simulink model "measurement_setup"  (R2021b)
settings: Solver=VariableStepAuto  StartTime=0.0  StopTime=sim_duration  MaxStep=1e-5  RelTol=1e-7
values from neighbouring files (symbols this model uses):
  f_gen = 6000    [amplitude_test_simulation.m]    (also in dibs_simulation.m; noise_simulation.m = params.generation_freq; prbs_simulation.m = 3000; simulate.m = params.generation_freq)
  Fs = 4*f_gen    (= 24000)    [amplitude_test_simulation.m]    (also in dibs_simulation.m; noise_simulation.m = params.sampling_freq; prbs_simulation.m = 12000; simulate.m = params.sampling_freq)
libraries: cstblocks x1
settings Model: Creator=stdnt  LastModifiedBy=stdnt
settings DataIOCC: ReturnWorkspaceOutputs=off

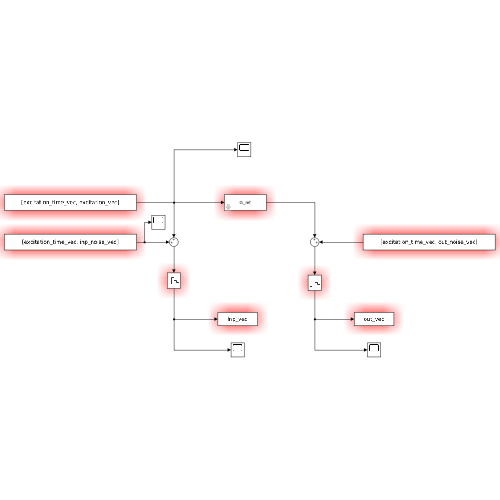
[thumbnail: Simulink's stored preview of the top-level diagram]
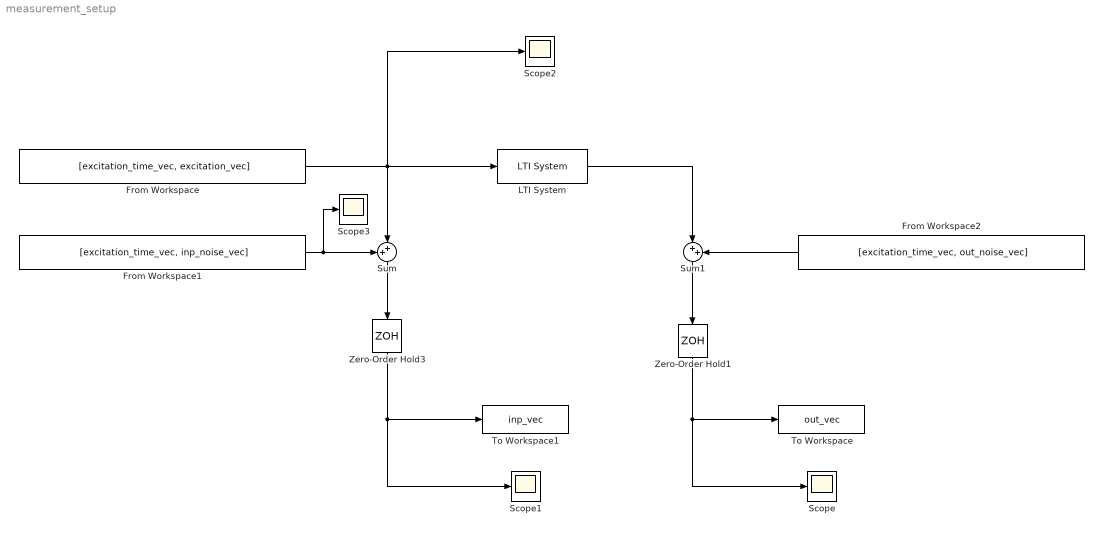
== system measurement_setup ==
  From Workspace : FromWorkspace  VariableName=[excitation_time_vec, excitation_vec]  SampleTime=1/f_gen  Interpolate=off  ZeroCross=off  OutputAfterFinalValue=Holding final value
  From Workspace1 : FromWorkspace  VariableName=[excitation_time_vec, inp_noise_vec]  SampleTime=1/f_gen  Interpolate=off  ZeroCross=off  OutputAfterFinalValue=Holding final value
  From Workspace2 : FromWorkspace  VariableName=[excitation_time_vec, out_noise_vec]  SampleTime=1/f_gen  Interpolate=off  ZeroCross=off  OutputAfterFinalValue=Holding final value
  LTI System : cstblocks/LTI System  sys=G_ref  IC=[]
  Scope{,1..3} (4 alike) : Scope
  Sum : Sum  Inputs=++|
  Sum1 : Sum  Inputs=|++
  To Workspace : ToWorkspace  VariableName=out_vec  SampleTime=1/Fs
  To Workspace1 : ToWorkspace  VariableName=inp_vec  SampleTime=1/Fs
  Zero-Order Hold1 : ZeroOrderHold  SampleTime=1/Fs
  Zero-Order Hold3 : ZeroOrderHold  SampleTime=1/Fs
  wires:
  Zero-Order Hold1/1 -> Scope/1, To Workspace/1
  Zero-Order Hold3/1 -> Scope1/1, To Workspace1/1
  From Workspace/1 -> Sum/2, Scope2/1, LTI System/1
  LTI System/1 -> Sum1/1
  Sum/1 -> Zero-Order Hold3/1
  Sum1/1 -> Zero-Order Hold1/1
  From Workspace1/1 -> Sum/1, Scope3/1
  From Workspace2/1 -> Sum1/2
